simulink model "simulateur_2D"  (R2019b)
settings: Solver=ode45  StartTime=0.0  StopTime=15  MaxStep=0.1  RelTol=1e-3  EnableMultiTasking=on
InitFcn:
  | % LRS TU KL %
  | % By Alen Turnwald %
  | % 09.01.2017 %
  | clc
  | close
  | 
  | %% g_q
  | g_q = [1;0];
  | 
  | 
  | if ~exist('mp','var')||~exist('mc','var')||~exist('L','var')||~exist('g','var')||~exist('d1','var')||~exist('d2','var')
  | % Model Paramter
  |     warning(['(Some) Model Parameter are not defined!' ,10, '****  Setting the predefined parameter  ****'])
  |     N = 2;
  |     mc = 1.5;
  |     mp = 0.5;
  |     g = 9.82;
  |     L = 1;
  | % Damping factors
  |     d1 = 1e-2;
  |     d2 = 1e-2;
  | end
  | 
  | if ~exist('x_0','var')
  | % Initial state
  |     warning(['(Initial state "x_0" not defined or wrongly named!' ,10, '****  Setting x_0 = [0.1; 10 deg; 0; 0]  ****'])
  |     x_0 = zeros(4,1);
  |     x_0(1) = 0.1;
  |     x_0(2) = 10*pi/180;
  | end
  | 
  | if ~exist('K_lqr','var')||~exist('Kd_lqr','var')
  |     warning(['(No controller found!' ,10, '****   Applying a predefined controller  ****'])
  |     K_lqr = [-14.1421  171.8846  -25.2787   54.7535];
  | end
StopFcn:
  | %% load data
  | 
  | load output
  | 
  | %% Read data
  | q1 = out.Data(:,1);
  | q2 = out.Data(:,2)*180/pi;
  | x_ref = out.Data(:,5);
  | t = out.Time;
  | 
  | 
  | %% Plot
  | % close all
  | figure(2)
  | clf
  | h(1) = subplot(2,1,1);
  | plot(t,q1,'b','LineWidth',2); grid on
  | 
  | hold on
  | plot(t,x_ref,'r--')
  | hold off
  | ylabel('q_1 [m]')
  | legend('q_1','q_1 ref')
  | 
  | h(2) = subplot(2,1,2);
  | plot(t,q2,'b','LineWidth',2); grid on
  | hold on
  | plot(t,zeros(1,length(t)),'r--')
  | hold off
  | ylabel('q_2 [°]')
  | legend('q_2','q_2 ref')
  | 
  | xlabel('t [s]')
  | 
  | linkaxes(h,'x')
undefined symbols (not defined in the file or in its folder): ki, Rroue
settings Model: Creator=Turnwald  LastModifiedBy=Gagey
settings DataIOCC: SaveFormat=Array  ReturnWorkspaceOutputs=off
settings OptimizationCC: OptimizeBlockIOStorage=off  BufferReuse=off  GlobalBufferReuse=off  ExpressionFolding=off  LocalBlockOutputs=off  LifeSpan=inf  OptimizeDataStoreBuffers=off  BusAssignmentInplaceUpdate=off
settings DebuggingCC: SolverPrmCheckMsg=warning  AllowSymbolicDim=off  SFUnexpectedBacktrackingDiag=warning  SFNoUnconditionalDefaultTransitionDiag=warning  SFExecutionAtInitializationDiag=none  ArithmeticOperatorsInVariantConditions=warning
settings HardwareCC: ProdBitPerPointer=32  ProdBitPerSizeT=32  ProdBitPerPtrDiffT=32  ProdLargestAtomicFloat=None  ProdIntDivRoundTo=Undefined  ProdEndianess=Unspecified  ProdWordSize=32  ProdHWDeviceType=32-bit Generic
settings ModelReferenceCC: PropagateSignalLabelsOutOfModel=off
settings SFSimCC: SimUseLocalCustomCode=off  CustomCodeUndefinedFunction=UseInterfaceOnly
settings RTWCC: RTWUseLocalCustomCode=off
settings CodeAppCC: StateflowObjectComments=on
settings GRTTargetCC: TargetLangStandard=C89/C90 (ANSI)  GeneratePreprocessorConditionals=Disable all
settings ConfigComp: CovMetricSettings=dw  CovHtmlReporting=on  CovSaveCumulativeToWorkspaceVar=on  CovSaveSingleToWorkspaceVar=on  CovExternalEMLEnable=off

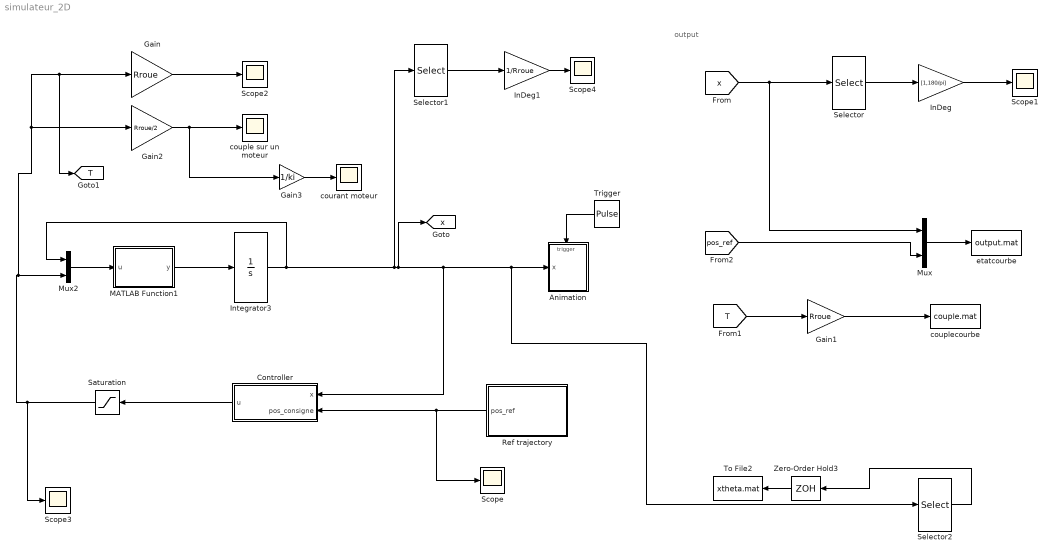
== system simulateur_2D ==
  note: output
  Animation : Subsystem
  Controller : Subsystem
  Gain : Gain  Gain=Rroue
  Gain1 : Gain  Gain=Rroue
  Gain2 : Gain  Gain=Rroue/2
  Gain3 : Gain  Gain=1/ki
  InDeg : Gain  Gain=[1,180/pi]
  InDeg1 : Gain  Gain=1/Rroue
  Integrator3 : Integrator  InitialCondition=[0;0.3;0;0]
  MATLAB Function1 : MATLAB Function  TreatAsAtomicUnit=on
  Mux : Mux  Inputs=2
  Mux2 : Mux  Inputs=2
  Ref trajectory : Subsystem
  Saturation : Saturate  UpperLimit=8  LowerLimit=-8
  Scope{,1..4} (5 alike) : Scope
  Selector : Selector  InputPortWidth=4  IndexOptions=Index vector (dialog)  Indices=[1:2]  OutputSizes=1
  Selector1 : Selector  InputPortWidth=4  IndexOptions=Index vector (dialog)  Indices=[3]  OutputSizes=1
  Selector2 : Selector  InputPortWidth=4  IndexOptions=Index vector (dialog)  Indices=[1,2]  OutputSizes=1
  To File2 : ToFile  Filename=xtheta.mat  SaveFormat=Timeseries  SampleTime=0.01
  Trigger : DiscretePulseGenerator  PulseType=Time based  Period=0.1  PulseWidth=50
  Zero-Order Hold3 : ZeroOrderHold  SampleTime=0.01
  couple sur un moteur : Scope
  couplecourbe : ToFile  Filename=couple.mat  MatrixName=coupleinput  SaveFormat=Timeseries
  courant moteur : Scope
  etatcourbe : ToFile  Filename=output.mat  MatrixName=out  SaveFormat=Timeseries
  tag scope: T=global, x=global
  wires:
  Ref trajectory/1(pos_ref) -> Scope/1, Controller/2(pos_consigne)
  MATLAB Function1/1(y) -> Integrator3/1
  Trigger/1 -> Animation/Trigger
  Integrator3/1 -> Selector2/1, Animation/1(x), Controller/1(x), [x], Selector1/1, Mux2/1
  Mux2/1 -> MATLAB Function1/1(u)
  [pos_ref] -> Mux/2
  Mux/1 -> etatcourbe/1
  Selector/1 -> InDeg/1
  InDeg/1 -> Scope1/1
  [x] -> Mux/1, Selector/1
  [T] -> Gain1/1
  Controller/1(u) -> Saturation/1
  Gain/1 -> Scope2/1
  Gain1/1 -> couplecourbe/1
  Gain2/1 -> Gain3/1, couple sur un moteur/1
  Gain3/1 -> courant moteur/1
  Saturation/1 -> Scope3/1, Gain2/1, [T], Gain/1, Mux2/2
  Selector1/1 -> InDeg1/1
  InDeg1/1 -> Scope4/1
  Zero-Order Hold3/1 -> To File2/1
  Selector2/1 -> Zero-Order Hold3/1

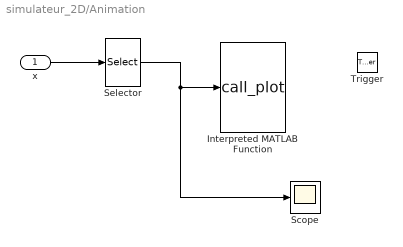
== system simulateur_2D/Animation ==
  x : Inport
  Trigger : TriggerPort  VariantControl=(inherit)  PortDimensions=1
  Interpreted MATLAB Function : MATLABFcn  MATLABFcn=call_plot  OutputDimensions=0
  Scope : Scope
  Selector : Selector  InputPortWidth=4  IndexOptions=Index vector (dialog)  Indices=[1:2]  OutputSizes=1
  wires:
  x/1 -> Selector/1
  Selector/1 -> Scope/1, Interpreted MATLAB Function/1

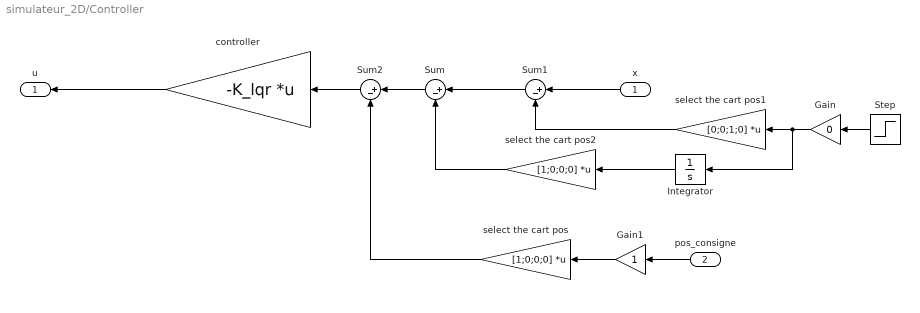
== system simulateur_2D/Controller ==
  x : Inport
  pos_consigne : Inport  Port=2
  Gain : Gain  Gain=0
  Gain1 : Gain
  Integrator : Integrator
  Step : Step  Time=10  Before=1  After=-1  SampleTime=0
  Sum : Sum  Inputs=|+-
  Sum1 : Sum  Inputs=|+-
  Sum2 : Sum  Inputs=|+-
  controller : Gain  Gain=-K_lqr  Multiplication=Matrix(K*u)
  select the cart pos : Gain  Gain=[1;0;0;0]  Multiplication=Matrix(K*u)
  select the cart pos1 : Gain  Gain=[0;0;1;0]  Multiplication=Matrix(K*u)
  select the cart pos2 : Gain  Gain=[1;0;0;0]  Multiplication=Matrix(K*u)
  u : Outport  VectorParamsAs1DForOutWhenUnconnected=off
  wires:
  controller/1 -> u/1
  Gain1/1 -> select the cart pos/1
  pos_consigne/1 -> Gain1/1
  x/1 -> Sum1/1
  Sum1/1 -> Sum/1
  select the cart pos1/1 -> Sum1/2
  Gain/1 -> Integrator/1, select the cart pos1/1
  Step/1 -> Gain/1
  select the cart pos2/1 -> Sum/2
  Integrator/1 -> select the cart pos2/1
  Sum/1 -> Sum2/1
  Sum2/1 -> controller/1
  select the cart pos/1 -> Sum2/2

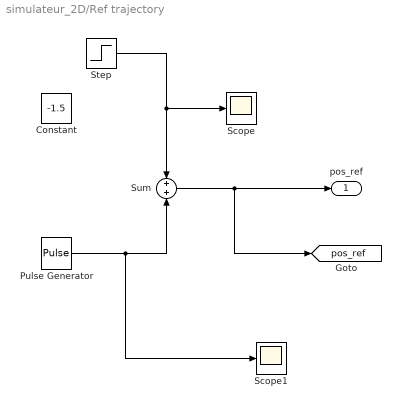
== system simulateur_2D/Ref trajectory ==
  Constant : Constant  Value=-1.5
  Pulse Generator : DiscretePulseGenerator  PulseType=Time based  Period=10  PulseWidth=50  PhaseDelay=2
  Scope : Scope
  Scope1 : Scope
  Step : Step  Time=2  After=-0.5  SampleTime=0
  Sum : Sum
  pos_ref : Outport  VectorParamsAs1DForOutWhenUnconnected=off
  tag scope: pos_ref=global
  wires:
  Sum/1 -> [pos_ref], pos_ref/1
  Pulse Generator/1 -> Scope1/1, Sum/2
  Step/1 -> Sum/1, Scope/1

== matlab function simulateur_2D/MATLAB Function1 ==
  data: u input; y output
function y = dynamique(u)
% fonction définissant la dynamique du système: renvoie f(X,U) avec X
% l'état, et U la variable de commande physique (composante T de la force
% appliquée au chariot)

x= u(1); %position linéaire roue
theta= u(2); %inclinaison du pendule
xdot= u(3); % vitesse linéaire roue
thetadot= u(4); % vitesse angulaire du pendule
T= u(5); % force (N) appliquée appliquée par lesmoteurs

% Defintion des paramètres du système
mr= 0.4; % masse roue + moteur
mp= 2; % masse pendule
l= 0.355; % longueur du pendule
%J=  m*l^2/3; % inertie du pendule
g= 9.81; % cste de gravité
d1= 0.2; % coeff. de frottement visqueux roue
d2= 0.1; % coeff. de frottement visqueux pendule

% Calcul des dérivées secondes
Matrice_masse=[mr+mp, -l*mp*cos(theta);-l*mp*cos(theta), l^2*mp];
Matrice_coriolis=[l*mp*thetadot^2*sin(theta);-l*g*mp*sin(theta)]+[d1*xdot;d2*thetadot];
C=[1;0];
xthetaddot=-inv(Matrice_masse)*Matrice_coriolis+inv(Matrice_masse)*C*T;
%Calcul de f
y = [xdot;thetadot;xthetaddot];
